simulink model "Berechnung_L_Model"  (Simulink 7.8)
settings: Solver=ode3  StartTime=0.0  StopTime=140*1e-3  FixedStep=1.4e-004  MaxStep=1e-6  RelTol=1e-6
undefined symbols (not defined in the file or in its folder): delta, FpyLookUp1, FpyLookUp2, KY1, KY2, Oy1, Oy2, Vy1, Vy2, yLookUp1, yLookUp2
libraries: simulink x1
settings Model: Creator=Markus  LastModifiedBy=Markus

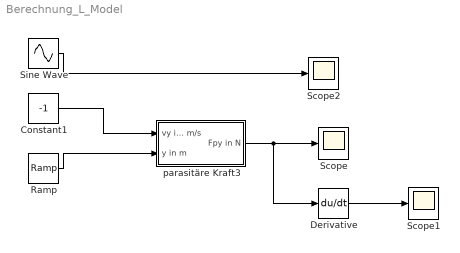
== system Berechnung_L_Model ==
  Constant1 : Constant  Value=-1
  Derivative : Derivative
  Ramp : simulink/Sources/Ramp  slope=1  start=0  X0=-70*1e-3
  Scope : Scope
      settings: YMin=-0.35  YMax=0.65  SaveName=Fx_minus_S
  Scope1 : Scope
      settings: YMin=-55000  YMax=55000
  Scope2 : Scope
      settings: YMin=5e-005  YMax=0.00045  SaveName=ScopeData2
  Sine Wave : Sin  Frequency=2*pi*0.1e3  SampleTime=0
  parasitäre Kraft3 : Subsystem
  wires:
  Ramp/1 -> parasitäre Kraft3/2(y in m)
  parasitäre Kraft3/1(Fpy in N) -> Scope/1, Derivative/1
  Derivative/1 -> Scope1/1
  Sine Wave/1 -> Scope2/1
  Constant1/1 -> parasitäre Kraft3/1(vy in m/s)

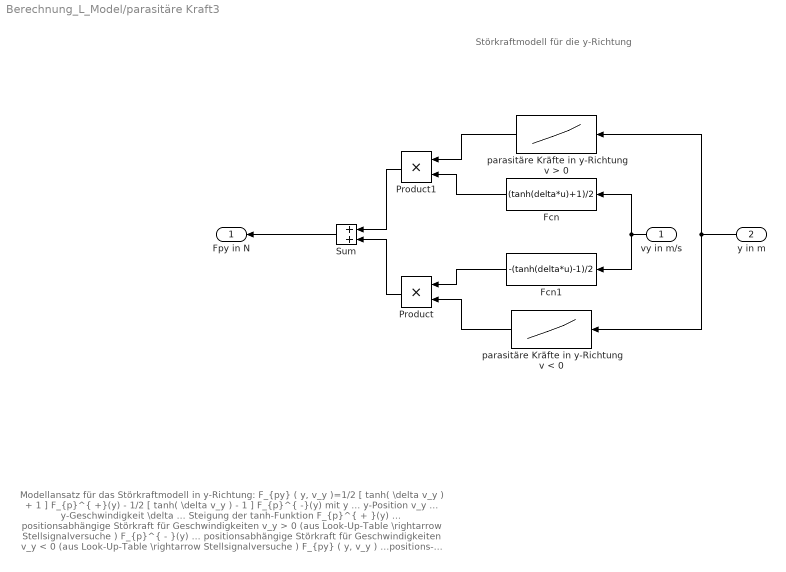
== system Berechnung_L_Model/parasitäre Kraft3 ==
  note: Störkraftmodell für die y-Richtung
  note: Modellansatz für das Störkraftmodell in y-Richtung:
      |
      | F_{py} ( y, v_y )=1/2 [ tanh(  \delta  v_y ) + 1 ] F_{p}^{  +}(y)  -  1/2 [ tanh( \delta  v_y )  - 1 ]  F_{p}^{  -}(y)
      |
      | mit
      |
      | y    ... y-Position
      | v_y  ... y-Geschwindigkeit
      | \delta   ... Steigung der tanh-Funktion
      |
      | F_{p}^{  + }(y)          ... positionsabhängige Störkraft für Geschwindigkeiten v_y   >  0  (aus Look-Up-Table \rightarrow Stellsignalversuche )
      | F_{p}^{  - }(y)           ... positionsabhängige Störkraft für Geschwindigkeiten v_y   <  0  (aus Look-Up-Table \rightarrow Stellsignalversuche )
      | F_{py} ( y, v_y ) ...positions- und richtungsabhängige Störkraft
  vy in m/s : Inport
  y in m : Inport  Port=2
  Fcn : Fcn  Expr=(tanh(delta*u)+1)/2
  Fcn1 : Fcn  Expr=-(tanh(delta*u)-1)/2
  Product : Product  RndMeth=Zero
  Product1 : Product  RndMeth=Zero
  Sum : Sum
  parasitäre Kräfte in y-Richtung v < 0 : Lookup_n-D  NumberOfTableDimensions=1  BreakpointsForDimension1=fliplr(yLookUp2')*1e-3+Vy2  Table=fliplr(FpyLookUp2')*KY2+Oy2  InterpMethod=Cubic spline  RndMeth=Simplest  InputSameDT=on
  parasitäre Kräfte in y-Richtung v > 0 : Lookup_n-D  NumberOfTableDimensions=1  BreakpointsForDimension1=yLookUp1*1e-3+Vy1  Table=FpyLookUp1*KY1+Oy1  InterpMethod=Cubic spline  RndMeth=Simplest  InputSameDT=on
  Fpy in N : Outport
  wires:
  parasitäre Kräfte in y-Richtung v < 0/1 -> Product/2
  parasitäre Kräfte in y-Richtung v > 0/1 -> Product1/1
  Product/1 -> Sum/2
  Product1/1 -> Sum/1
  Fcn/1 -> Product1/2
  Fcn1/1 -> Product/1
  Sum/1 -> Fpy in N/1
  vy in m/s/1 -> Fcn/1, Fcn1/1
  y in m/1 -> parasitäre Kräfte in y-Richtung v > 0/1, parasitäre Kräfte in y-Richtung v < 0/1
